simulink model "DigitalControlsProject"  (R2017a)
settings: Solver=VariableStepAuto  StartTime=0.0  StopTime=10.0  RelTol=1e-3
undefined symbols (not defined in the file or in its folder): modelD
settings Model: Creator=windo  LastModifiedBy=Alphakyl

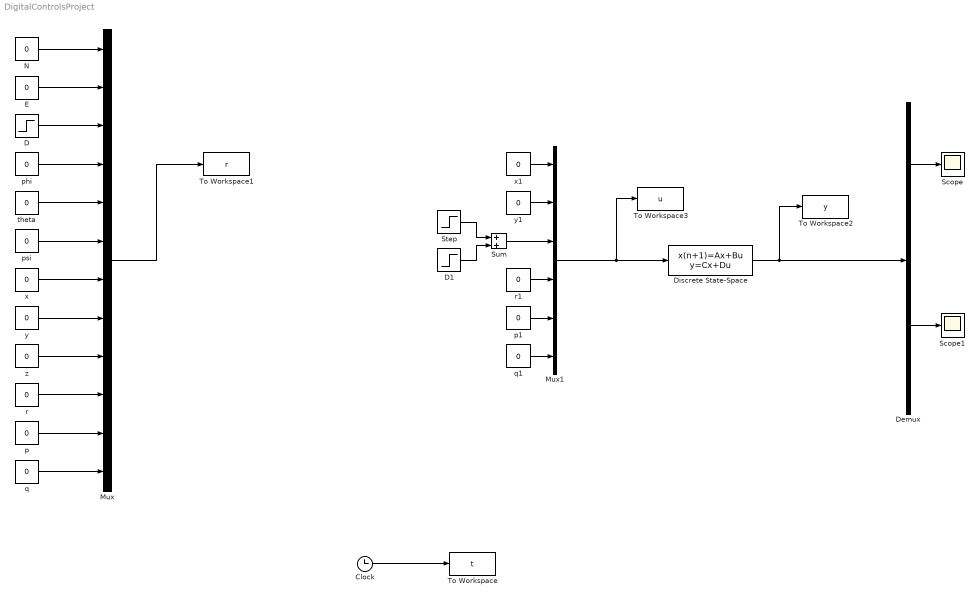
== system DigitalControlsProject ==
  Clock : Clock
  D : Step  SampleTime=0
  D1 : Step  SampleTime=0
  Demux : Demux  Outputs=12
  Discrete State-Space : DiscreteStateSpace  A=modelD.A  B=modelD.B  C=modelD.C  D=modelD.D  SampleTime=-1
  E : Constant  Value=0
  Mux : Mux  Inputs=12
  Mux1 : Mux  Inputs=6
  N : Constant  Value=0
  Scope : Scope
  Scope1 : Scope
  Step : Step  Time=4  Before=1  After=0  SampleTime=0
  Sum : Sum
  To Workspace : ToWorkspace  VariableName=t  SampleTime=-1
  To Workspace1 : ToWorkspace  VariableName=r  SampleTime=-1
  To Workspace2 : ToWorkspace  VariableName=y  SampleTime=-1
  To Workspace3 : ToWorkspace  VariableName=u  SampleTime=-1
  p : Constant  Value=0
  p1 : Constant  Value=0
  phi : Constant  Value=0
  psi : Constant  Value=0
  q : Constant  Value=0
  q1 : Constant  Value=0
  r : Constant  Value=0
  r1 : Constant  Value=0
  theta : Constant  Value=0
  x : Constant  Value=0
  x1 : Constant  Value=0
  y : Constant  Value=0
  y1 : Constant  Value=0
  z : Constant  Value=0
  wires:
  Mux1/1 -> To Workspace3/1, Discrete State-Space/1
  Clock/1 -> To Workspace/1
  Mux/1 -> To Workspace1/1
  D/1 -> Mux/3
  N/1 -> Mux/1
  phi/1 -> Mux/4
  theta/1 -> Mux/5
  psi/1 -> Mux/6
  x/1 -> Mux/7
  y/1 -> Mux/8
  z/1 -> Mux/9
  r/1 -> Mux/10
  p/1 -> Mux/11
  q/1 -> Mux/12
  E/1 -> Mux/2
  x1/1 -> Mux1/1
  q1/1 -> Mux1/6
  p1/1 -> Mux1/5
  r1/1 -> Mux1/4
  y1/1 -> Mux1/2
  Step/1 -> Sum/1
  D1/1 -> Sum/2
  Sum/1 -> Mux1/3
  Discrete State-Space/1 -> Demux/1, To Workspace2/1
  Demux/3 -> Scope/1
  Demux/9 -> Scope1/1
